simulink model "ej7_2"  (R2023a)
settings: Solver=VariableStepAuto  StartTime=0.0  StopTime=30  MaxStep=1e-4  RelTol=1e-3
settings Model: Creator=Juan  LastModifiedBy=Juan

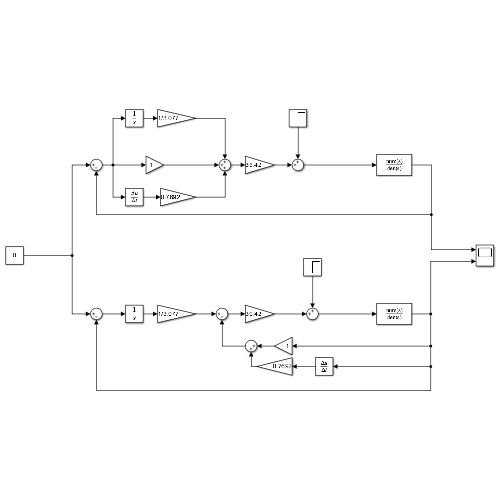
[thumbnail: Simulink's stored preview of the top-level diagram]
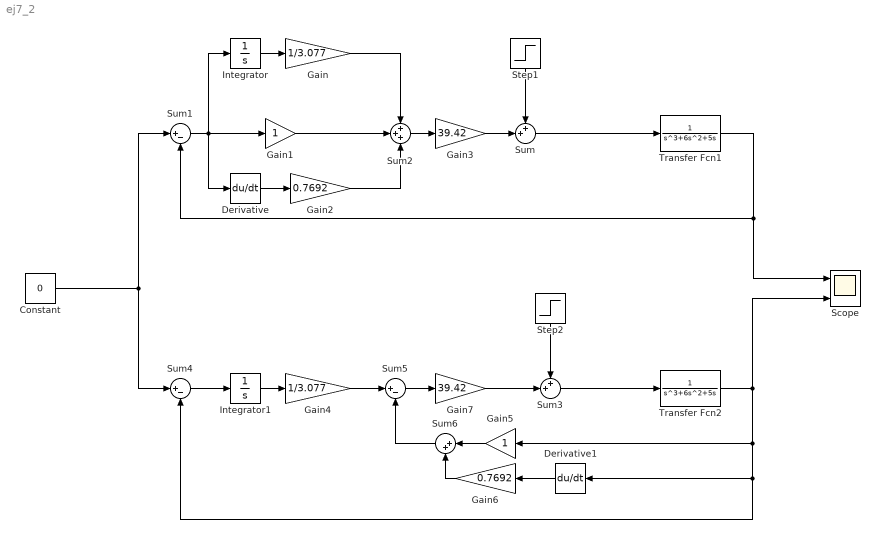
== system ej7_2 ==
  Constant : Constant  Value=0
  Derivative : Derivative
  Derivative1 : Derivative
  Gain : Gain  Gain=1/3.077
  Gain1 : Gain
  Gain2 : Gain  Gain=0.7692
  Gain3 : Gain  Gain=39.42
  Gain4 : Gain  Gain=1/3.077
  Gain5 : Gain
  Gain6 : Gain  Gain=0.7692
  Gain7 : Gain  Gain=39.42
  Integrator : Integrator
  Integrator1 : Integrator
  Scope : Scope  NumInputPorts=2
  Step1 : Step  After=10  SampleTime=0
  Step2 : Step  After=10  SampleTime=0
  Sum : Sum  Inputs=++|
  Sum1 : Sum  Inputs=|+-
  Sum2 : Sum  Inputs=+++
  Sum3 : Sum  Inputs=++|
  Sum4 : Sum  Inputs=|+-
  Sum5 : Sum  Inputs=|+-
  Sum6 : Sum  Inputs=|++
  Transfer Fcn1 : TransferFcn  Numerator=[ 1 ]  Denominator=[ 1 6 5 0]
  Transfer Fcn2 : TransferFcn  Numerator=[ 1 ]  Denominator=[ 1 6 5 0]
  wires:
  Sum/1 -> Transfer Fcn1/1
  Transfer Fcn1/1 -> Scope/1, Sum1/2
  Constant/1 -> Sum4/1, Sum1/1
  Step1/1 -> Sum/1
  Sum1/1 -> Derivative/1, Gain1/1, Integrator/1
  Integrator/1 -> Gain/1
  Gain/1 -> Sum2/1
  Sum2/1 -> Gain3/1
  Gain1/1 -> Sum2/2
  Derivative/1 -> Gain2/1
  Gain2/1 -> Sum2/3
  Gain3/1 -> Sum/2
  Integrator1/1 -> Gain4/1
  Sum4/1 -> Integrator1/1
  Step2/1 -> Sum3/1
  Transfer Fcn2/1 -> Scope/2, Gain5/1, Derivative1/1, Sum4/2
  Sum3/1 -> Transfer Fcn2/1
  Gain7/1 -> Sum3/2
  Gain4/1 -> Sum5/1
  Sum5/1 -> Gain7/1
  Gain5/1 -> Sum6/1
  Sum6/1 -> Sum5/2
  Gain6/1 -> Sum6/2
  Derivative1/1 -> Gain6/1
